simulink model "gimbal_control_22b"  (R2022b)
settings: Solver=VariableStepAuto  StartTime=0.0  StopTime=10.0  RelTol=1e-3
InitFcn:
  | init
undefined symbols (not defined in the file or in its folder): pa
settings Model: Creator=Administrator  LastModifiedBy=HQ03
settings SolverCC: AlgebraicLoopSolver=TrustRegion
settings OptimizationCC: ReuseModelBlockBuffer=on
settings DebuggingCC: UnconnectedInputMsg=warning  UnconnectedOutputMsg=warning  UnconnectedLineMsg=warning
settings ModelReferenceCC: EnableRefExpFcnMdlSchedulingChecks=on

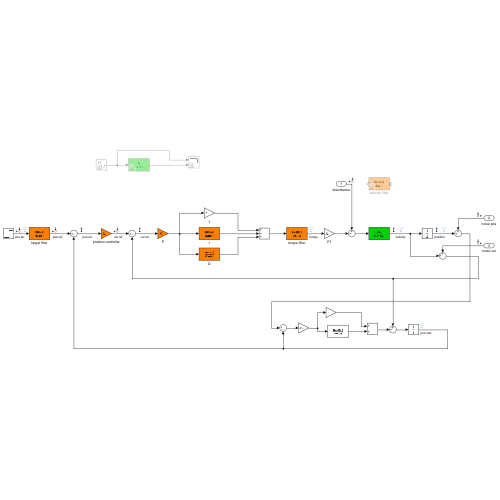
[thumbnail: Simulink's stored preview of the top-level diagram]
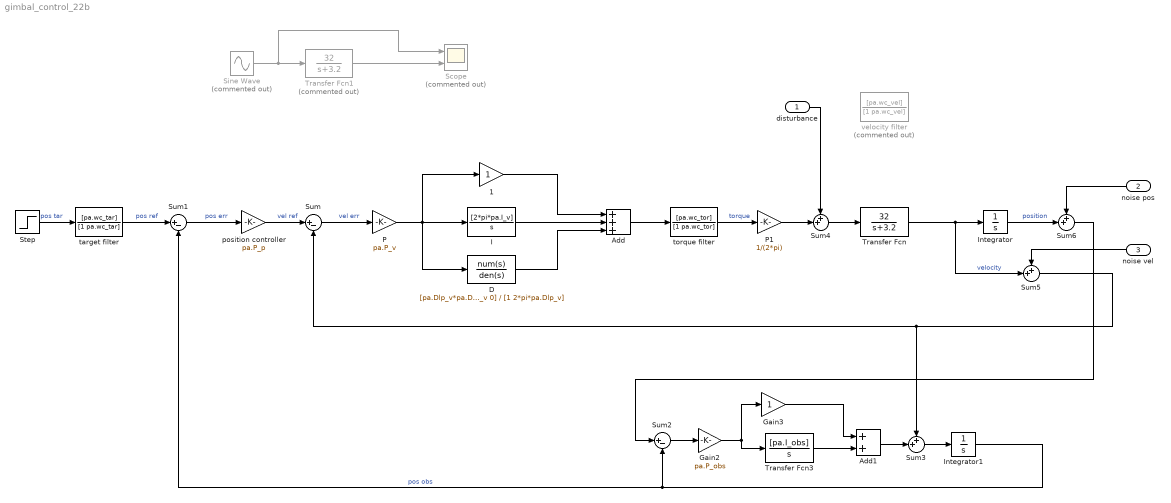
== system gimbal_control_22b ==
  disturbance : Inport
  noise pos : Inport  Port=2
  noise vel : Inport  Port=3
  1 : Gain
  Add : Sum  Inputs=+++
  Add1 : Sum
  D : TransferFcn  Numerator=[pa.Dlp_v*pa.D_v 0]  Denominator=[1 2*pi*pa.Dlp_v]
  Gain2 : Gain  Gain=pa.P_obs
  Gain3 : Gain
  I : TransferFcn  Numerator=[2*pi*pa.I_v]  Denominator=[1 0]
  Integrator : Integrator
  Integrator1 : Integrator
  P : Gain  Gain=pa.P_v
  P1 : Gain  Gain=1/(2*pi)
  Scope : Scope  Commented=on  NumInputPorts=2
  Sine Wave : Sin  Commented=on  Frequency=2*pi  SampleTime=0
  Step : Step  SampleTime=0
  Sum : Sum  Inputs=|+-
  Sum1 : Sum  Inputs=|+-
  Sum2 : Sum  Inputs=|+-
  Sum{3..6} (4 alike) : Sum  Inputs=++|
  Transfer Fcn : TransferFcn  Numerator=[32]  Denominator=[1 3.2]
  Transfer Fcn1 : TransferFcn  Commented=on  Numerator=[32]  Denominator=[1 3.2]
  Transfer Fcn3 : TransferFcn  Numerator=[pa.I_obs]  Denominator=[1 0]
  position controller : Gain  Gain=pa.P_p
  target filter : TransferFcn  Numerator=[pa.wc_tar]  Denominator=[1 pa.wc_tar]
  torque filter : TransferFcn  Numerator=[pa.wc_tor]  Denominator=[1 pa.wc_tor]
  velocity filter : TransferFcn  Commented=on  Numerator=[pa.wc_vel]  Denominator=[1 pa.wc_vel]
  wires:
  Transfer Fcn/1 -> Integrator/1, Sum5/2  "velocity"
  Sum/1 -> P/1  "vel err"
  position controller/1 -> Sum/1  "vel ref"
  Sum1/1 -> position controller/1  "pos err"
  Step/1 -> target filter/1  "pos tar"
  target filter/1 -> Sum1/1  "pos ref"
  Sum2/1 -> Gain2/1
  Add1/1 -> Sum3/2
  Sum3/1 -> Integrator1/1
  Integrator1/1 -> Sum2/2, Sum1/2  "pos obs"
  Sum4/1 -> Transfer Fcn/1
  Add/1 -> torque filter/1
  disturbance/1 -> Sum4/1
  Integrator/1 -> Sum6/2  "position"
  noise pos/1 -> Sum6/1
  noise vel/1 -> Sum5/1
  Sum6/1 -> Sum2/1
  P/1 -> D/1, I/1, 1/1
  1/1 -> Add/1
  I/1 -> Add/2
  D/1 -> Add/3
  Gain2/1 -> Transfer Fcn3/1, Gain3/1
  Gain3/1 -> Add1/1
  Transfer Fcn3/1 -> Add1/2
  Sum5/1 -> Sum/2, Sum3/1
  P1/1 -> Sum4/2
  Transfer Fcn1/1 -> Scope/2
  Sine Wave/1 -> Scope/1, Transfer Fcn1/1
  torque filter/1 -> P1/1  "torque"
